simulink model "lab2"  (R2019b)
settings: Solver=FixedStepAuto  StartTime=0.0  StopTime=0.05  FixedStep=0.0001  RelTol=1e-3
libraries: powerlib x22, powerlib_meascontrol x5, simulink_extras x3
settings Model: Creator=100448597  LastModifiedBy=robom
settings DataIOCC: SaveOutput=off  ReturnWorkspaceOutputs=off
settings SFSimCC: CustomCodeUndefinedFunction=UseInterfaceOnly

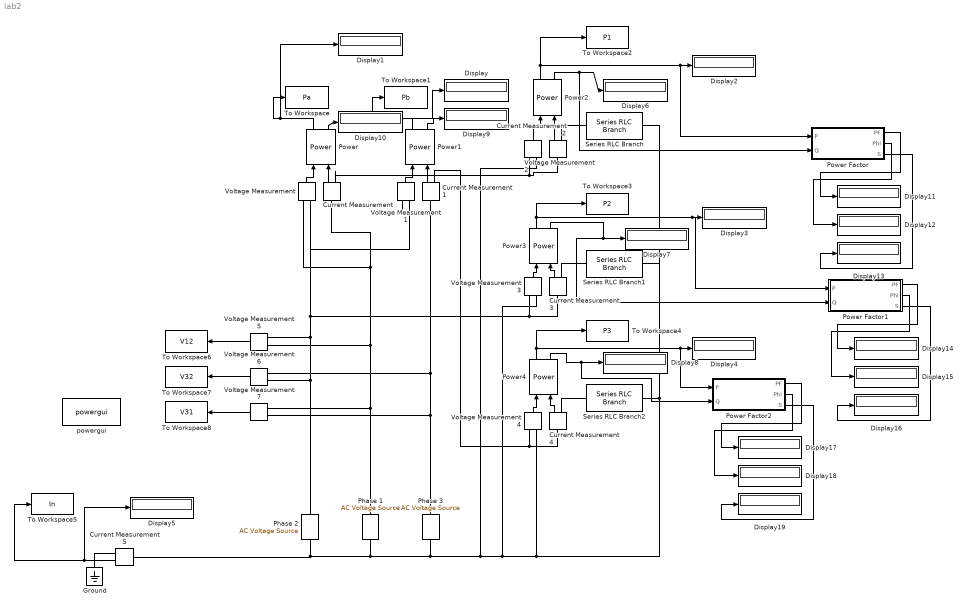
== system lab2 ==
  Current Measurement{,1..5} (6 alike) : powerlib/Measurements/Current Measurement  PhasorSimulation=off  OutputType=Complex  PSBequivalent=0
      settings: SourceProductName=Simscape Electrical
  Display{,1..19} (20 alike) : Display
  Ground : powerlib/Elements/Ground  LConnTagsString=a
      settings: SourceProductName=Simscape Electrical
  Phase 1 : powerlib/Electrical Sources/AC Voltage Source  Amplitude=330  Phase=0  Frequency=50  SampleTime=0  Measurements=None  BusType=swing  Pref=10e3  Qref=0  Qmin=-inf  Qmax=+inf
      settings: SourceProductName=Simscape Electrical
  Phase 2 : powerlib/Electrical Sources/AC Voltage Source  Amplitude=330  Phase=-120  Frequency=50  SampleTime=0  Measurements=None  BusType=swing  Pref=10e3  Qref=0  Qmin=-inf  Qmax=+inf
      settings: SourceProductName=Simscape Electrical
  Phase 3 : powerlib/Electrical Sources/AC Voltage Source  Amplitude=330  Phase=120  Frequency=50  SampleTime=0  Measurements=None  BusType=swing  Pref=10e3  Qref=0  Qmin=-inf  Qmax=+inf
      settings: SourceProductName=Simscape Electrical
  Power : powerlib_meascontrol/Measurements/Power  Freq=50  Vinit=[1, 0]  Iinit=[1, 0]  Ts=0
      settings: SourceProductName=Simscape Electrical
  Power Factor : Subsystem
  Power Factor1 : Subsystem
  Power Factor2 : Subsystem
  Power{1..4} (4 alike) : powerlib_meascontrol/Measurements/Power  Freq=50  Vinit=[0, 0]  Iinit=[0, 0]  Ts=0
      settings: SourceProductName=Simscape Electrical
  Series RLC Branch : powerlib/Elements/Series RLC Branch  LConnTagsString=__new0  RConnTagsString=__new0  BranchType=RLC  Resistance=125  Inductance=0  SetiL0=off  InitialCurrent=0  Capacitance=0  Setx0=off  InitialVoltage=0  Measurements=None
      settings: SourceProductName=Simscape Electrical
  Series RLC Branch1 : powerlib/Elements/Series RLC Branch  LConnTagsString=__new0  RConnTagsString=__new0  BranchType=RLC  Resistance=125  Inductance=0  SetiL0=off  InitialCurrent=0  Capacitance=0  Setx0=off  InitialVoltage=0  Measurements=None
      settings: SourceProductName=Simscape Electrical
  Series RLC Branch2 : powerlib/Elements/Series RLC Branch  LConnTagsString=__new0  RConnTagsString=__new0  BranchType=RLC  Resistance=125  Inductance=0  SetiL0=off  InitialCurrent=0  Capacitance=0  Setx0=off  InitialVoltage=0  Measurements=None
      settings: SourceProductName=Simscape Electrical
  To Workspace : ToWorkspace  VariableName=Pa  SampleTime=-1
      settings: Save2DSignal=2-D array (concatenate along first dimension)
  To Workspace1 : ToWorkspace  VariableName=Pb  SampleTime=-1
      settings: Save2DSignal=2-D array (concatenate along first dimension)
  To Workspace2 : ToWorkspace  VariableName=P1  SampleTime=-1
      settings: Save2DSignal=2-D array (concatenate along first dimension)
  To Workspace3 : ToWorkspace  VariableName=P2  SampleTime=-1
      settings: Save2DSignal=2-D array (concatenate along first dimension)
  To Workspace4 : ToWorkspace  VariableName=P3  SampleTime=-1
      settings: Save2DSignal=2-D array (concatenate along first dimension)
  To Workspace5 : ToWorkspace  VariableName=In  SampleTime=-1
      settings: Save2DSignal=2-D array (concatenate along first dimension)
  To Workspace6 : ToWorkspace  VariableName=V12  SampleTime=-1
      settings: Save2DSignal=2-D array (concatenate along first dimension)
  To Workspace7 : ToWorkspace  VariableName=V32  SampleTime=-1
      settings: Save2DSignal=2-D array (concatenate along first dimension)
  To Workspace8 : ToWorkspace  VariableName=V31  SampleTime=-1
      settings: Save2DSignal=2-D array (concatenate along first dimension)
  Voltage Measurement{,1..7} (8 alike) : powerlib/Measurements/Voltage Measurement  PhasorSimulation=off  OutputType=Complex  PSBequivalent=0
      settings: SourceProductName=Simscape Electrical
  powergui : powerlib/powergui  Priority=1  SimulationMode=Continuous  SampleTime=50e-6  frequency=60  Iterations=50  frequencyindice=50  Pbase=100e6  ErrMax=1e-4  UnitsV=kV  UnitsW=MW  buscounter=0  FunctionMessages=off  echomessages=off  EnableUseOfTLC=off  CurrentSourceSwitches=off  DisableSnubberDevices=off  DisableRonSwitches=off  DisableVfSwitches=off  DisplayEquations=off  AutomaticDiscreteSolvers=off  SolverType=Tustin/Backward Euler (TBE)  Interpol=off  ExternalGateDelay=off  methode=off  Ts=100  x0status=blocks  SPID=on  SwTol=0  HookPort=off  NonlinearTolerance=0  nMaxIteration=15  ContinueOnMaxIteration=off  RestoreLinks=warning  ResistiveCurrentMeasurement=off  Frange=[0:2:500]  Ylog=off  Xlog=on  ShowGrid=off  save=off  variable=ZData  structure=0  ZoomFFT=off  StartTime=0.0  cycles=1  DisplayStyle=1  fundamental=60  FreqAxis=off  MaxFrequency=1000  frequencyindicesteady=1  RmsSteady=1  display=off
      settings: SourceProductName=Simscape Electrical
  wires:
  Voltage Measurement/1 -> Power/1
  Current Measurement/1 -> Power/2
  Power/1 -> To Workspace/1, Display1/1
  Power1/1 -> To Workspace1/1, Display/1
  Current Measurement1/1 -> Power1/2
  Voltage Measurement1/1 -> Power1/1
  Voltage Measurement2/1 -> Power2/1
  Current Measurement2/1 -> Power2/2
  Current Measurement3/1 -> Power3/2
  Voltage Measurement3/1 -> Power3/1
  Power3/1 -> To Workspace3/1, Power Factor1/1(P), Display3/1
  Voltage Measurement4/1 -> Power4/1
  Current Measurement4/1 -> Power4/2
  Current Measurement5/1 -> To Workspace5/1, Display5/1
  Voltage Measurement5/1 -> To Workspace6/1
  Voltage Measurement6/1 -> To Workspace7/1
  Voltage Measurement7/1 -> To Workspace8/1
  Power2/1 -> Power Factor/1(P), Display2/1, To Workspace2/1
  Power4/1 -> To Workspace4/1, Power Factor2/1(P), Display4/1
  Power2/2 -> Power Factor/2(Q), Display6/1
  Power3/2 -> Display7/1, Power Factor1/2(Q)
  Power4/2 -> Power Factor2/2(Q), Display8/1
  Power1/2 -> Display9/1
  Power/2 -> Display10/1
  Power Factor/1(PF) -> Display11/1
  Power Factor/3(S) -> Display13/1
  Power Factor/2(Phi) -> Display12/1
  Power Factor1/3(S) -> Display16/1
  Power Factor1/1(PF) -> Display14/1
  Power Factor1/2(Phi) -> Display15/1
  Power Factor2/3(S) -> Display19/1
  Power Factor2/1(PF) -> Display17/1
  Power Factor2/2(Phi) -> Display18/1
  connections:
  Current Measurement2/RConn1 -- Series RLC Branch/LConn1
  Current Measurement3/RConn1 -- Series RLC Branch1/LConn1
  Current Measurement4/RConn1 -- Series RLC Branch2/LConn1
  Phase 2/LConn1 -- Series RLC Branch/RConn1 -- Series RLC Branch1/RConn1 -- Series RLC Branch2/RConn1 -- Voltage Measurement4/LConn2 -- Voltage Measurement3/LConn2 -- Voltage Measurement2/LConn2 -- Phase 3/LConn1 -- Phase 1/LConn1 -- Current Measurement5/LConn1
  Current Measurement5/RConn1 -- Ground/LConn1
  Current Measurement/LConn1 -- Voltage Measurement/LConn1 -- Voltage Measurement5/LConn2 -- Voltage Measurement7/LConn1 -- Phase 1/RConn1
  Current Measurement/RConn1 -- Voltage Measurement2/LConn1 -- Current Measurement2/LConn1
  Current Measurement3/LConn1 -- Voltage Measurement3/LConn1 -- Voltage Measurement1/LConn2 -- Voltage Measurement/LConn2 -- Voltage Measurement5/LConn1 -- Voltage Measurement6/LConn2 -- Phase 2/RConn1
  Phase 3/RConn1 -- Voltage Measurement7/LConn2 -- Voltage Measurement6/LConn1 -- Voltage Measurement1/LConn1 -- Current Measurement1/LConn1
  Current Measurement1/RConn1 -- Voltage Measurement4/LConn1 -- Current Measurement4/LConn1

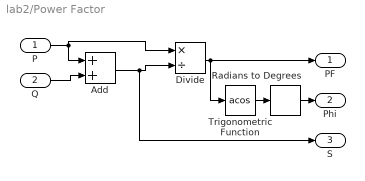
== system lab2/Power Factor ==
  P : Inport
  Q : Inport  Port=2
  Add : Sum
  Divide : Product  Inputs=*/
  Radians to Degrees : simulink_extras/Transformations/Radians to Degrees
  Trigonometric Function : Trigonometry  Operator=acos
  PF : Outport
  Phi : Outport  Port=2
  S : Outport  Port=3
  wires:
  Q/1 -> Add/2
  P/1 -> Add/1, Divide/1
  Add/1 -> S/1, Divide/2
  Divide/1 -> PF/1, Trigonometric Function/1
  Trigonometric Function/1 -> Radians to Degrees/1
  Radians to Degrees/1 -> Phi/1

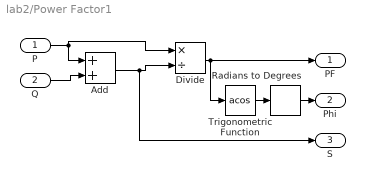
== system lab2/Power Factor1 ==
  P : Inport
  Q : Inport  Port=2
  Add : Sum
  Divide : Product  Inputs=*/
  Radians to Degrees : simulink_extras/Transformations/Radians to Degrees
  Trigonometric Function : Trigonometry  Operator=acos
  PF : Outport
  Phi : Outport  Port=2
  S : Outport  Port=3
  wires:
  Q/1 -> Add/2
  P/1 -> Add/1, Divide/1
  Add/1 -> S/1, Divide/2
  Divide/1 -> PF/1, Trigonometric Function/1
  Trigonometric Function/1 -> Radians to Degrees/1
  Radians to Degrees/1 -> Phi/1

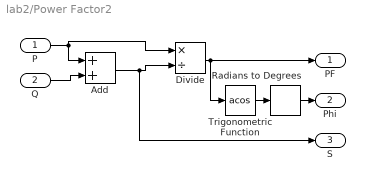
== system lab2/Power Factor2 ==
  P : Inport
  Q : Inport  Port=2
  Add : Sum
  Divide : Product  Inputs=*/
  Radians to Degrees : simulink_extras/Transformations/Radians to Degrees
  Trigonometric Function : Trigonometry  Operator=acos
  PF : Outport
  Phi : Outport  Port=2
  S : Outport  Port=3
  wires:
  Q/1 -> Add/2
  P/1 -> Add/1, Divide/1
  Add/1 -> S/1, Divide/2
  Divide/1 -> PF/1, Trigonometric Function/1
  Trigonometric Function/1 -> Radians to Degrees/1
  Radians to Degrees/1 -> Phi/1
